simulink model "pacemaker_top"  (R2024b)
settings: Solver=FixedStepDiscrete  StartTime=0.0  StopTime=1  FixedStep=1e-3  RelTol=1e-3
undefined symbols (not defined in the file): A0, A1, PTB2, PTB3
libraries: frdmk64flib x4, etargetslib x2
settings Model: ExtModeTrigDuration=5  Creator=marwa  LastModifiedBy=habel
settings OptimizationCC: DefaultParameterBehavior=Inlined  EnhancedBackFolding=on  PassReuseOutputArgsAs=Individual arguments  ZeroExternalMemoryAtStartup=off  ZeroInternalMemoryAtStartup=off  MaxStackSize=64  OptimizeBlockOrder=speed  DifferentSizesBufferReuse=on  OptimizationCustomize=off  EfficientTunableParamExpr=on
settings DebuggingCC: ParameterTunabilityLossMsg=error
settings HardwareCC: ProdBitPerPointer=32  ProdBitPerSizeT=32  ProdBitPerPtrDiffT=32  ProdLargestAtomicInteger=Long  ProdLargestAtomicFloat=Double  ProdWordSize=32  ProdHWDeviceType=ARM Compatible->ARM Cortex
settings SFSimCC: MATLABDynamicMemAlloc=off
settings RTWCC: Description=Embedded Coder  SystemTargetFile=ert.tlc  HardwareBoard=NXP FRDM-K64F  TLCOptions="-aInlineSetEventsForThisBaseRateFcn=TLC_FALSE -aSuppressMultiTaskScheduler=TLC_FALSE  -aRateBasedStepFcn=0"  TemplateMakefile=ert_default_tmf  Toolchain=GNU Tools for ARM Embedded Processors
settings CodeAppCC: ForceParamTrailComments=on  IgnoreCustomStorageClasses=off  OperatorAnnotations=on  SimulinkDataObjDesc=on  SFDataObjDesc=on  InsertBlockDesc=on
settings ERTTargetCC: ExtModeTransport=4  ExtModeMexFile=sendToCommService

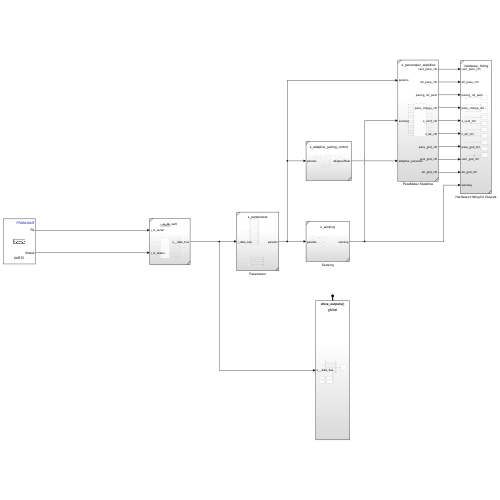
[thumbnail: Simulink's stored preview of the top-level diagram]
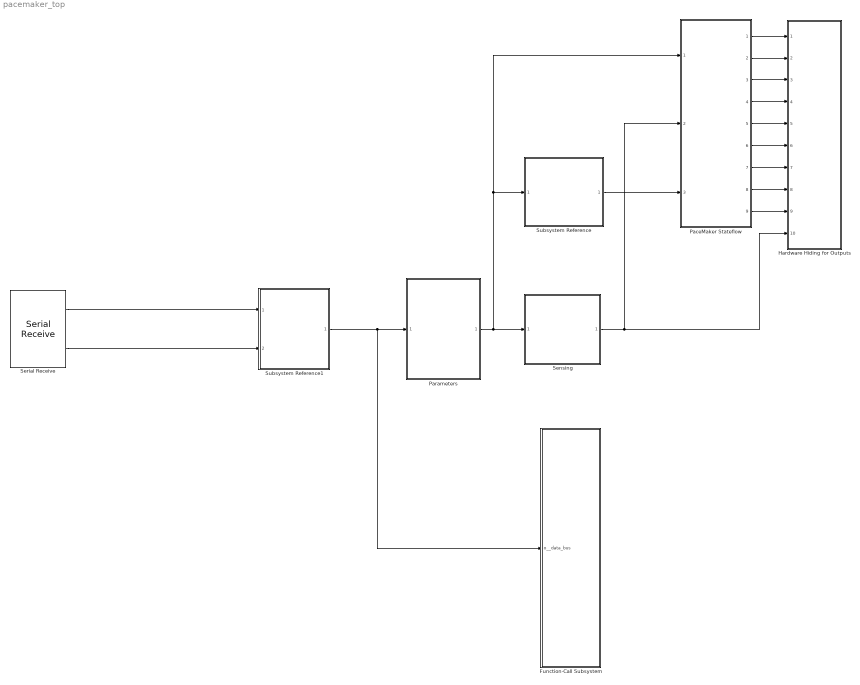
== system pacemaker_top ==
  Function-Call Subsystem : Subsystem  TreatAsAtomicUnit=on
  Hardware Hiding for Outputs : Subsystem  ReferencedSubsystem=hardware_hiding
  PaceMaker Stateflow : Subsystem  ReferencedSubsystem=s_pacemaker_stateflow
  Parameters : Subsystem  ReferencedSubsystem=s_parameters
  Sensing : Subsystem  ReferencedSubsystem=s_sensing
  Serial Receive : frdmk64flib/Serial Receive  SCIModule=0  Baudrate=uint32(9600)  Parity=None  StopBits=1  HardwareFlowControl=None  ByteOrder=LittleEndian  DataType=uint8  DataLength=16  BlockingMode=off  OutputStatus=on  SampleTime=0.001
  Subsystem Reference : Subsystem  ReferencedSubsystem=s_adaptive_pacing_control
  Subsystem Reference1 : Subsystem  ReferencedSubsystem=s_rx_uart
      settings: MinAlgLoopOccurrences=on
  wires:
  Parameters/1 -> Sensing/1, PaceMaker Stateflow/1, Subsystem Reference/1
  Sensing/1 -> PaceMaker Stateflow/2, Hardware Hiding for Outputs/10
  PaceMaker Stateflow/1 -> Hardware Hiding for Outputs/1
  PaceMaker Stateflow/2 -> Hardware Hiding for Outputs/2
  PaceMaker Stateflow/3 -> Hardware Hiding for Outputs/3
  PaceMaker Stateflow/4 -> Hardware Hiding for Outputs/4
  PaceMaker Stateflow/5 -> Hardware Hiding for Outputs/5
  PaceMaker Stateflow/6 -> Hardware Hiding for Outputs/6
  PaceMaker Stateflow/7 -> Hardware Hiding for Outputs/7
  PaceMaker Stateflow/8 -> Hardware Hiding for Outputs/8
  PaceMaker Stateflow/9 -> Hardware Hiding for Outputs/9
  Subsystem Reference1/1 -> Function-Call Subsystem/1(o__data_bus), Parameters/1
  Subsystem Reference/1 -> PaceMaker Stateflow/3
  Serial Receive/1 -> Subsystem Reference1/1
  Serial Receive/2 -> Subsystem Reference1/2

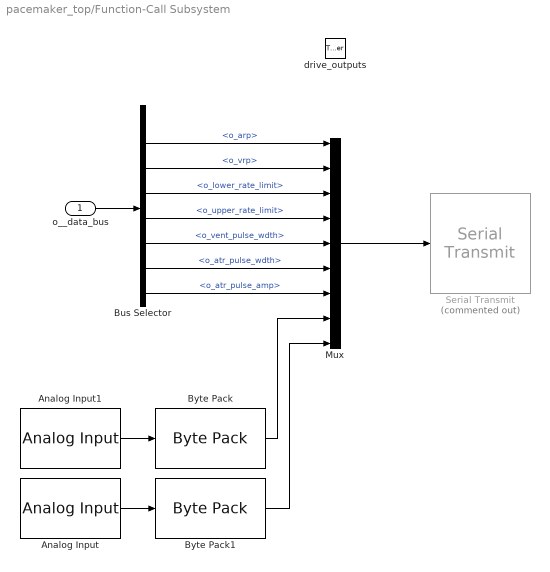
== system pacemaker_top/Function-Call Subsystem ==
  o__data_bus : Inport
  drive_outputs : TriggerPort  TriggerType=function-call  IsSimulinkFunction=on  FunctionName=drive_outputs  VariantControl=(inherit)
  Analog Input : frdmk64flib/Analog Input  Whichpin=PTB3 (A1)  SampleTime=-1
  Analog Input1 : frdmk64flib/Analog Input  Whichpin=PTB2 (A0)  SampleTime=-1
  Bus Selector : BusSelector  OutputSignals=o_mode,o_arp,o_vrp,o_lower_rate_limit,o_upper_rate_limit,o_vent_pulse_wdth,o_atr_pulse_wdth,o_atr_pulse_amp
  Byte Pack : etargetslib/Byte Pack  datatypes={'double'}  byteAlign=1
  Byte Pack1 : etargetslib/Byte Pack  datatypes={'double'}  byteAlign=1
  Mux : Mux  Inputs=9
  Serial Transmit : frdmk64flib/Serial Transmit  Commented=on  SCIModule=0  Baudrate=uint32(9600)  Parity=None  StopBits=1  HardwareFlowControl=None  ByteOrder=LittleEndian  BlockingMode=on  OutputStatus=off
  wires:
  Mux/1 -> Serial Transmit/1
  o__data_bus/1 -> Bus Selector/1
  Analog Input/1 -> Byte Pack1/1
  Bus Selector/5 -> Mux/4  "<o_upper_rate_limit>"
  Bus Selector/8 -> Mux/7  "<o_atr_pulse_amp>"
  Byte Pack1/1 -> Mux/9
  Bus Selector/3 -> Mux/2  "<o_vrp>"
  Bus Selector/7 -> Mux/6  "<o_atr_pulse_wdth>"
  Byte Pack/1 -> Mux/8
  Bus Selector/2 -> Mux/1  "<o_arp>"
  Bus Selector/6 -> Mux/5  "<o_vent_pulse_wdth>"
  Bus Selector/4 -> Mux/3  "<o_lower_rate_limit>"
  Analog Input1/1 -> Byte Pack/1
